simulink model "Motor"  (R2014a)
settings: Solver=ode45  StartTime=0.0  StopTime=10  MaxStep=1  RelTol=1e-3
model workspace: external: MAT-File EMRAX_228HV.mat (data not in the file)
undefined symbols (not defined in the file or in its folder): eta, Ld, Lq, phi_m, R
settings Model: Creator=abk  LastModifiedBy=Nathan
settings DataIOCC: ExternalInput=Is omega  LoadExternalInput=on

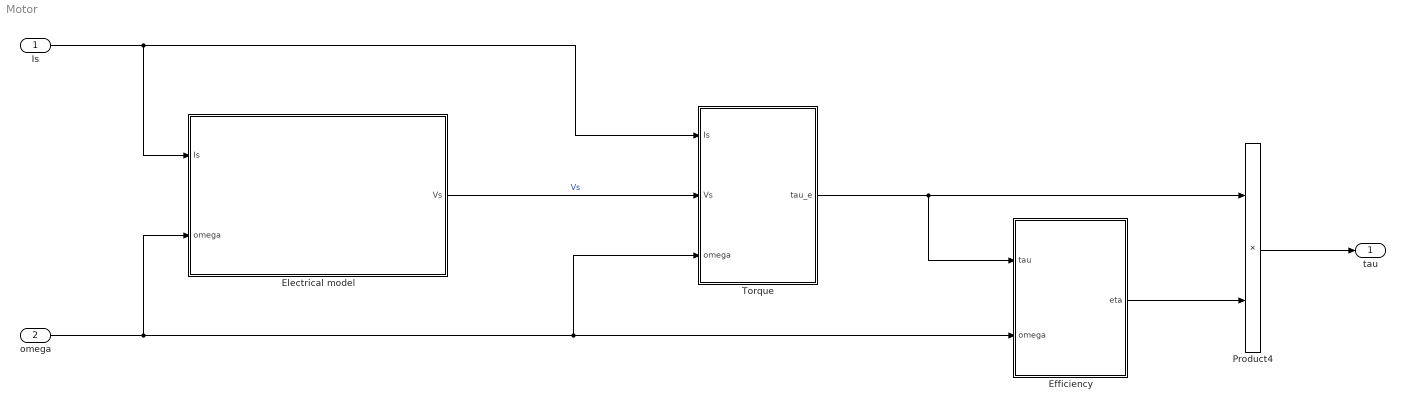
== system Motor ==
  Is : Inport  OutDataTypeStr=Bus: Is_bus
  omega : Inport  Port=2
  Efficiency : Subsystem
  Electrical model : Subsystem
  Product4 : Product
  Torque : Subsystem
  tau : Outport
  wires:
  omega/1 -> Electrical model/2(omega), Torque/3(omega), Efficiency/2(omega)
  Is/1 -> Electrical model/1(Is), Torque/1(Is)
  Electrical model/1(Vs) -> Torque/2(Vs)  "Vs"
  Torque/1(tau_e) -> Efficiency/1(tau), Product4/1
  Efficiency/1(eta) -> Product4/2
  Product4/1 -> tau/1

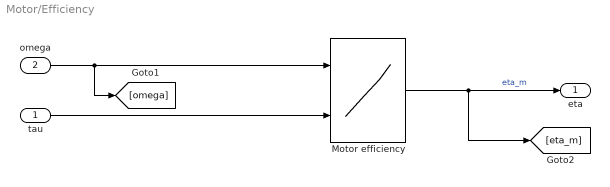
== system Motor/Efficiency ==
  tau : Inport
  omega : Inport  Port=2
  Motor efficiency : Lookup_n-D  BreakpointsForDimension1=eta.speed  BreakpointsForDimension2=eta.tau  Table=eta.eta  InternalRulePriority=Speed  RndMeth=Simplest  InputSameDT=on
  eta : Outport
  wires:
  omega/1 -> Motor efficiency/1, [omega]
  Motor efficiency/1 -> eta/1, [eta_m]  "eta_m"
  tau/1 -> Motor efficiency/2

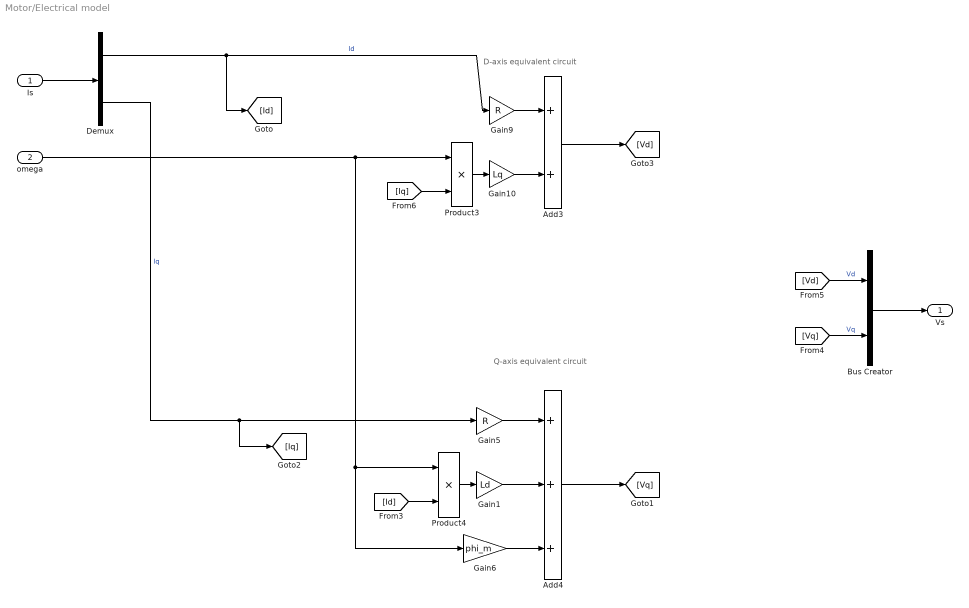
== system Motor/Electrical model ==
  note: D-axis equivalent circuit
  note: Q-axis equivalent circuit
  Is : Inport
  omega : Inport  Port=2
  Add3 : Sum
  Add4 : Sum  Inputs=+++
  Bus Creator : BusCreator  Inputs='Vd','Vq'
  Demux : Demux  Outputs=2
  Gain1 : Gain  Gain=Ld
  Gain10 : Gain  Gain=Lq
  Gain5 : Gain  Gain=R
  Gain6 : Gain  Gain=phi_m
  Gain9 : Gain  Gain=R
  Product3 : Product
  Product4 : Product
  Vs : Outport
  wires:
  Gain9/1 -> Add3/1
  [Iq] -> Product3/2
  Product3/1 -> Gain10/1
  omega/1 -> Gain6/1, Product4/1, Product3/1
  Gain10/1 -> Add3/2
  Add3/1 -> [Vd]
  Gain6/1 -> Add4/3
  [Id] -> Product4/2
  Product4/1 -> Gain1/1
  Gain1/1 -> Add4/2
  Gain5/1 -> Add4/1
  Demux/2 -> [Iq], Gain5/1  "Iq"
  Add4/1 -> [Vq]
  Is/1 -> Demux/1
  Demux/1 -> [Id], Gain9/1  "Id"
  [Vd] -> Bus Creator/1  "Vd"
  [Vq] -> Bus Creator/2  "Vq"
  Bus Creator/1 -> Vs/1

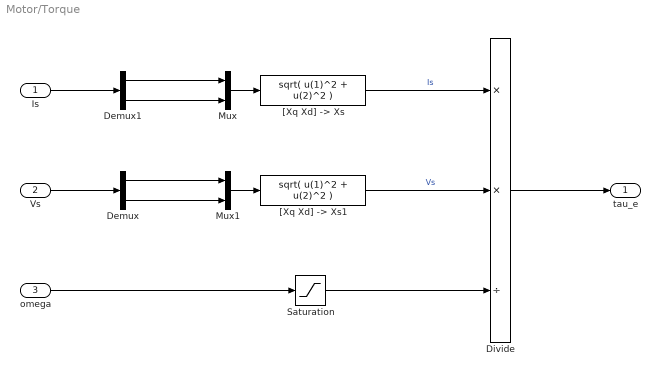
== system Motor/Torque ==
  Is : Inport
  Vs : Inport  Port=2
  omega : Inport  Port=3
  Demux : Demux  Outputs=2
  Demux1 : Demux  Outputs=2
  Divide : Product  Inputs=**/
  Mux : Mux  Inputs=2
  Mux1 : Mux  Inputs=2
  Saturation : Saturate  UpperLimit=inf  LowerLimit=0.1
  "[Xq Xd] -> Xs" : Fcn  Expr=sqrt( u(1)^2 + u(2)^2 )
  "[Xq Xd] -> Xs1" : Fcn  Expr=sqrt( u(1)^2 + u(2)^2 )
  tau_e : Outport
  wires:
  Is/1 -> Demux1/1
  Demux1/1 -> Mux/1
  Demux1/2 -> Mux/2
  Mux/1 -> "[Xq Xd] -> Xs"/1
  "[Xq Xd] -> Xs"/1 -> Divide/1  "Is"
  Mux1/1 -> "[Xq Xd] -> Xs1"/1
  Demux/1 -> Mux1/1
  Demux/2 -> Mux1/2
  Vs/1 -> Demux/1
  "[Xq Xd] -> Xs1"/1 -> Divide/2  "Vs"
  omega/1 -> Saturation/1
  Divide/1 -> tau_e/1
  Saturation/1 -> Divide/3
